simulink model "controller_model"  (R2024a)
settings: Solver=VariableStepAuto  StartTime=0.0  StopTime=4.0  MaxStep=1e-6  RelTol=1e-6  AbsTol=1e-6  EnableMultiTasking=on
values from neighbouring files (symbols this model uses):
  D = 2 * zeta * w_n * J_e    (= 0.0031028075591)    [controller_parameters.m]    (also in main.m = 2 * zeta * w_n * J_e; main_feedforward.m = 2 * zeta * w_n * J_e)
  J_e = (J_m + J_r/N^2)    (= 1.64609053498e-05)    [controller_parameters.m]    (also in main.m = (J_mr + J_r); main_feedforward.m = (J_mr + J_r))
  K_e = K_r /N    [controller_parameters.m]    (also in main.m = angular_spring_constant; main_feedforward.m = angular_spring_constant)
  N = 36    [controller_parameters.m]    (also in generateMotorDataFromFile.m = size(M, 1); generateMotorDataFromTrajFile.m = size(M, 1); main.m; main_feedforward.m = 9)
  P = w_n^2 * J_e - K_e    [controller_parameters.m]    (also in main.m; main_feedforward.m)
  w_f = w_n *10    (= 942.477796077)    [controller_parameters.m]    (also in main.m = 837.758040957; main_feedforward.m = 837.758040957)
settings Model: Creator=james  LastModifiedBy=james
settings SolverCC: AutoScaleAbsTol=off  AlgebraicLoopSolver=TrustRegion  MaxZcPerStep=1
settings DataIOCC: LimitDataPoints=on  MaxDataPoints=10000
settings OptimizationCC: ReuseModelBlockBuffer=off  LifeSpan=inf
settings DebuggingCC: UnconnectedInputMsg=warning  UnconnectedOutputMsg=warning  UnconnectedLineMsg=warning  AllowSymbolicDim=off  SubsystemReferenceDiagnosticForUnitTest=warning  SFUnexpectedBacktrackingDiag=warning  SFNoUnconditionalDefaultTransitionDiag=warning  SFExecutionAtInitializationDiag=none  ArithmeticOperatorsInVariantConditions=warning
settings ModelReferenceCC: EnableRefExpFcnMdlSchedulingChecks=on
settings SFSimCC: SimUseLocalCustomCode=off  CustomCodeUndefinedFunction=UseInterfaceOnly
settings RTWCC: RTWUseLocalCustomCode=off  GPUComputeCapability=3.5  DLArmComputeVersion=19.05
settings CodeAppCC: StateflowObjectComments=on
settings GRTTargetCC: TargetLangStandard=C89/C90 (ANSI)
settings ConfigComp: CovMetricSettings=dw  CovSaveCumulativeToWorkspaceVar=on  CovSaveSingleToWorkspaceVar=on  CovExternalEMLEnable=off  CovSFcnEnable=off
settings SimscapeCC: SimscapeLogType=all  SimscapeLogSimulationStatistics=on  SimscapeLogDataHistory=10000

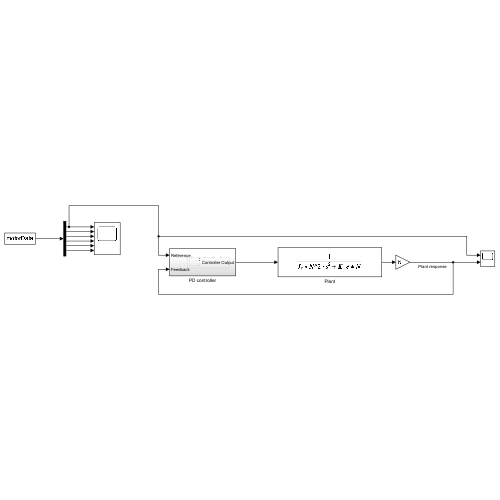
[thumbnail: Simulink's stored preview of the top-level diagram]
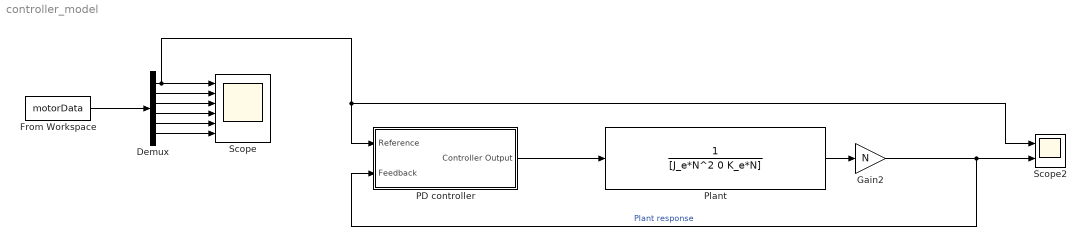
== system controller_model ==
  Demux : Demux  Outputs=6
  From Workspace : FromWorkspace  VariableName=motorData
  Gain2 : Gain  Gain=N
  PD controller : Subsystem
  Plant : TransferFcn  Denominator=[J_e*N^2 0 K_e*N]
  Scope : Scope  NumInputPorts=6
  Scope2 : Scope  NumInputPorts=2
  wires:
  From Workspace/1 -> Demux/1
  Demux/2 -> Scope/2
  Demux/3 -> Scope/3
  Demux/4 -> Scope/4
  Demux/5 -> Scope/5
  Demux/6 -> Scope/6
  Gain2/1 -> PD controller/2(Feedback), Scope2/2  "Plant response"
  PD controller/1(Controller Output) -> Plant/1
  Demux/1 -> Scope2/1, PD controller/1(Reference), Scope/1
  Plant/1 -> Gain2/1

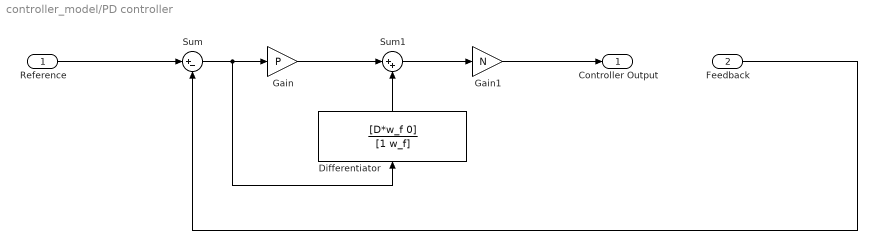
== system controller_model/PD controller ==
  Reference : Inport
  Feedback : Inport  Port=2
  Differentiator : TransferFcn  Numerator=[D*w_f 0]  Denominator=[1 w_f]
  Gain : Gain  Gain=P
  Gain1 : Gain  Gain=N
  Sum : Sum  Inputs=|+-
  Sum1 : Sum  Inputs=|++
  Controller Output : Outport
  wires:
  Sum/1 -> Differentiator/1, Gain/1
  Gain1/1 -> Controller Output/1
  Sum1/1 -> Gain1/1
  Differentiator/1 -> Sum1/2
  Feedback/1 -> Sum/2
  Gain/1 -> Sum1/1
  Reference/1 -> Sum/1
